simulink model "CL2CM1"  (R2024a)
settings: Solver=VariableStepAuto  StartTime=0.0  StopTime=10.0  RelTol=1e-3
settings Model: Creator=jeonghyun  LastModifiedBy=gluts

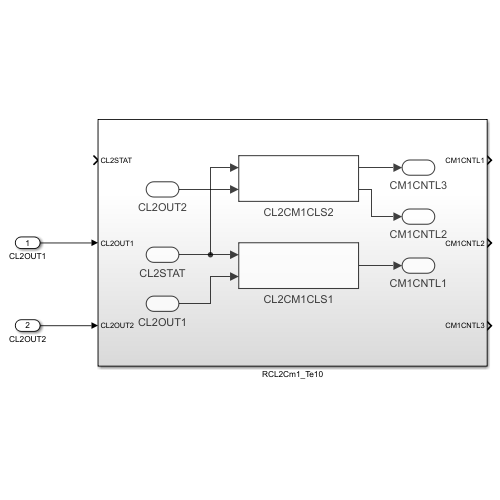
[thumbnail: Simulink's stored preview of the top-level diagram]
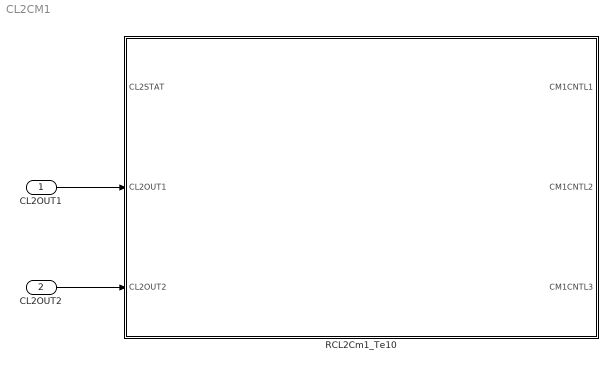
== system CL2CM1 ==
  CL2OUT1 : Inport
  CL2OUT2 : Inport  Port=2
  RCL2Cm1_Te10 : Subsystem
  wires:
  CL2OUT1/1 -> RCL2Cm1_Te10/2(CL2OUT1)
  CL2OUT2/1 -> RCL2Cm1_Te10/3(CL2OUT2)

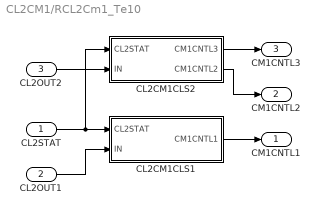
== system CL2CM1/RCL2Cm1_Te10 ==
  CL2STAT : Inport
  CL2OUT1 : Inport  Port=2
  CL2OUT2 : Inport  Port=3
  CL2CM1CLS1 : Subsystem
  CL2CM1CLS2 : Subsystem
  CM1CNTL1 : Outport
  CM1CNTL2 : Outport  Port=2
  CM1CNTL3 : Outport  Port=3
  wires:
  CL2OUT1/1 -> CL2CM1CLS1/2(IN)
  CL2STAT/1 -> CL2CM1CLS2/1(CL2STAT), CL2CM1CLS1/1(CL2STAT)
  CL2OUT2/1 -> CL2CM1CLS2/2(IN)
  CL2CM1CLS2/1(CM1CNTL3) -> CM1CNTL3/1
  CL2CM1CLS2/2(CM1CNTL2) -> CM1CNTL2/1
  CL2CM1CLS1/1(CM1CNTL1) -> CM1CNTL1/1

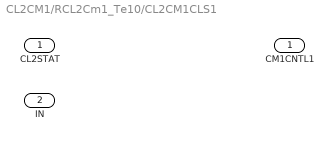
== system CL2CM1/RCL2Cm1_Te10/CL2CM1CLS1 ==
  CL2STAT : Inport
  IN : Inport  Port=2
  CM1CNTL1 : Outport

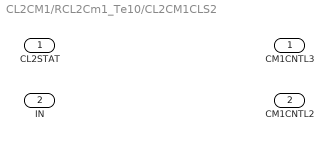
== system CL2CM1/RCL2Cm1_Te10/CL2CM1CLS2 ==
  CL2STAT : Inport
  IN : Inport  Port=2
  CM1CNTL3 : Outport
  CM1CNTL2 : Outport  Port=2
